simulink model "control"  (R2017a)
settings: Solver=ode4  StartTime=0.0  StopTime=100  FixedStep=0.01  RelTol=1e-3
values from neighbouring files (symbols this model uses):
  xnc = fac .* Op(i, :) + x    [Inv.m]    (also in gen.m = son)
undefined symbols (not defined in the file or in its folder): A, B, C, D
settings Model: Creator=aposad31  LastModifiedBy=santiago

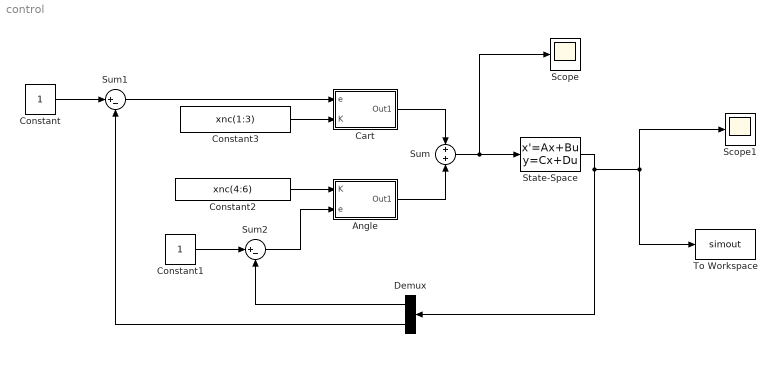
== system control ==
  Angle : Subsystem
  Cart : Subsystem
  Constant : Constant
  Constant1 : Constant
  Constant2 : Constant  Value=xnc(4:6)  VectorParams1D=off
  Constant3 : Constant  Value=xnc(1:3)
  Demux : Demux  Outputs=2
  Scope : Scope
  Scope1 : Scope
  State-Space : StateSpace  A=A  B=B  C=C  D=D  X0=0
  Sum : Sum
  Sum1 : Sum  Inputs=|+-
  Sum2 : Sum  Inputs=|+-
  To Workspace : ToWorkspace  VariableName=simout  SampleTime=-1
  wires:
  Constant3/1 -> Cart/2(K)
  Constant2/1 -> Angle/1(K)
  Angle/1(Out1) -> Sum/2
  Cart/1(Out1) -> Sum/1
  Demux/2 -> Sum1/2
  Constant/1 -> Sum1/1
  Sum1/1 -> Cart/1(e)
  Demux/1 -> Sum2/2
  Constant1/1 -> Sum2/1
  Sum2/1 -> Angle/2(e)
  Sum/1 -> Scope/1, State-Space/1
  State-Space/1 -> Demux/1, To Workspace/1, Scope1/1

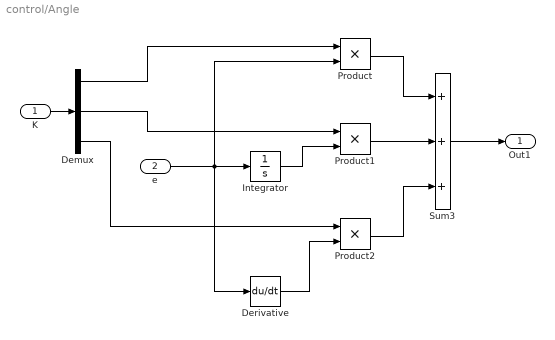
== system control/Angle ==
  K : Inport
  e : Inport  Port=2
  Demux : Demux  Outputs=3
  Derivative : Derivative
  Integrator : Integrator
  Product : Product
  Product1 : Product
  Product2 : Product
  Sum3 : Sum  Inputs=+++
  Out1 : Outport
  wires:
  Sum3/1 -> Out1/1
  Derivative/1 -> Product2/2
  e/1 -> Derivative/1, Product/2, Integrator/1
  Demux/1 -> Product/1
  Demux/2 -> Product1/1
  Integrator/1 -> Product1/2
  Demux/3 -> Product2/1
  Product2/1 -> Sum3/3
  Product1/1 -> Sum3/2
  Product/1 -> Sum3/1
  K/1 -> Demux/1

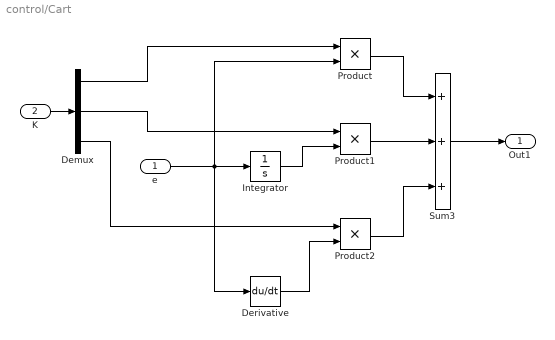
== system control/Cart ==
  e : Inport
  K : Inport  Port=2
  Demux : Demux  Outputs=3
  Derivative : Derivative
  Integrator : Integrator
  Product : Product
  Product1 : Product
  Product2 : Product
  Sum3 : Sum  Inputs=+++
  Out1 : Outport
  wires:
  Sum3/1 -> Out1/1
  Derivative/1 -> Product2/2
  e/1 -> Derivative/1, Product/2, Integrator/1
  Demux/1 -> Product/1
  Demux/2 -> Product1/1
  Integrator/1 -> Product1/2
  Demux/3 -> Product2/1
  Product2/1 -> Sum3/3
  Product1/1 -> Sum3/2
  Product/1 -> Sum3/1
  K/1 -> Demux/1
